simulink library "ctrl_ADRC_TD"  (R2018b)
settings: Solver=VariableStepAuto  StartTime=0.0  StopTime=10.0  RelTol=1e-3
settings Model: Creator=Huitao Lv  LastModifiedBy=Huitao Lv

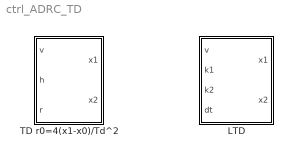
== system ctrl_ADRC_TD ==
  LTD : Subsystem  mask(LTD){}
      mask help: 线性跟踪微分器
  TD r0=4(x1-x0)/Td^2 : Subsystem  mask(TD){}
      mask help: 非线性跟踪微分器

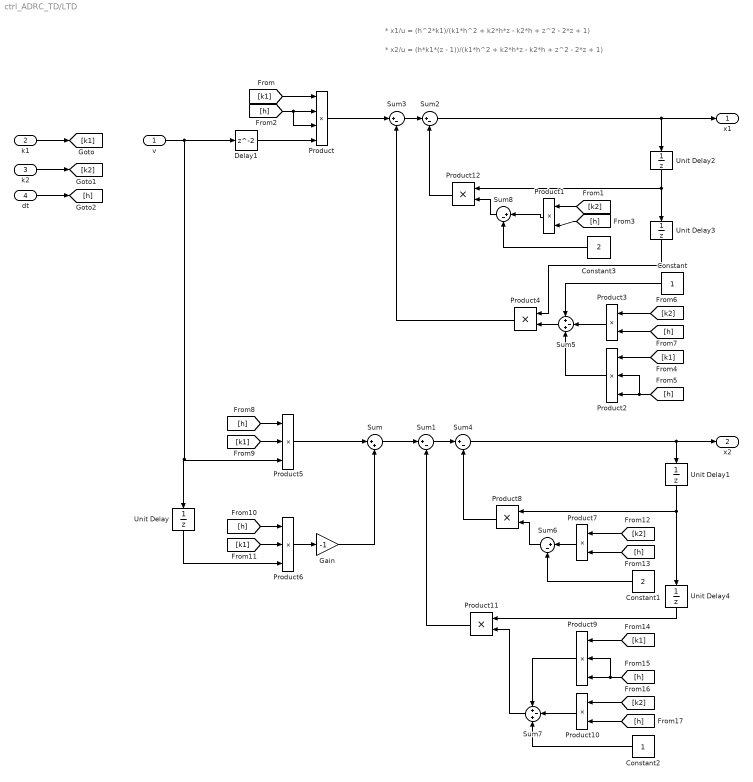
== system ctrl_ADRC_TD/LTD ==
  note: * x1/u = (h^2*k1)/(k1*h^2 + k2*h*z - k2*h + z^2 - 2*z + 1)
  note: * x2/u = (h*k1*(z - 1))/(k1*h^2 + k2*h*z - k2*h + z^2 - 2*z + 1)
  v : Inport
  k1 : Inport  Port=2
  k2 : Inport  Port=3
  dt : Inport  Port=4
  Constant : Constant  OutDataTypeStr=single
  Constant1 : Constant  Value=2  OutDataTypeStr=single
  Constant2 : Constant  OutDataTypeStr=single
  Constant3 : Constant  Value=2  OutDataTypeStr=single
  Delay1 : Delay
  Gain : Gain  Gain=-1
      settings: AttributesFormatString=%<Gain>
  Product : Product  Inputs=4
  Product1 : Product  Inputs=**
  Product{3..4,7..8,10..12} (7 alike) : Product
  Product{2,5..6,9} (4 alike) : Product  Inputs=3
  Sum : Sum  Inputs=|++
  Sum{1..4,6,8} (6 alike) : Sum  Inputs=|+-
  Sum5 : Sum  Inputs=+-+
  Sum7 : Sum  Inputs=+-+
  Unit Delay{,1..4} (5 alike) : UnitDelay  SampleTime=-1
  x1 : Outport
  x2 : Outport  Port=2
  wires:
  Constant3/1 -> Sum8/2
  Sum8/1 -> Product12/2
  Unit Delay2/1 -> Unit Delay3/1, Product12/1
  Product12/1 -> Sum2/2
  Product1/1 -> Sum8/1
  [k2] -> Product1/1
  Sum2/1 -> Unit Delay2/1, x1/1
  Unit Delay4/1 -> Product11/1
  Gain/1 -> Sum/2
  Product/1 -> Sum3/1
  Sum3/1 -> Sum2/1
  Unit Delay3/1 -> Product4/1
  Product8/1 -> Sum4/2
  Product4/1 -> Sum3/2
  v/1 -> Delay1/1, Product5/3, Unit Delay/1
  Unit Delay1/1 -> Unit Delay4/1, Product8/1
  Product5/1 -> Sum/1
  Sum/1 -> Sum1/1
  Delay1/1 -> Product/4
  Sum1/1 -> Sum4/1
  Sum4/1 -> x2/1, Unit Delay1/1
  Product11/1 -> Sum1/2
  dt/1 -> [h]
  k2/1 -> [k2]
  k1/1 -> [k1]
  [k1] -> Product/1
  [h] -> Product/3, Product/2
  [h] -> Product1/2
  [k1] -> Product2/1
  [h] -> Product2/2, Product2/3
  [k2] -> Product3/1
  [h] -> Product3/2
  Product2/1 -> Sum5/3
  Product3/1 -> Sum5/2
  Constant/1 -> Sum5/1
  Sum5/1 -> Product4/2
  [h] -> Product5/1
  [k1] -> Product5/2
  [k1] -> Product6/2
  [h] -> Product6/1
  Product6/1 -> Gain/1
  Unit Delay/1 -> Product6/3
  [k2] -> Product7/1
  [h] -> Product7/2
  Product7/1 -> Sum6/1
  Constant1/1 -> Sum6/2
  Sum6/1 -> Product8/2
  [h] -> Product9/3, Product9/2
  [k1] -> Product9/1
  Product9/1 -> Sum7/1
  Product10/1 -> Sum7/2
  [h] -> Product10/2
  [k2] -> Product10/1
  Constant2/1 -> Sum7/3
  Sum7/1 -> Product11/2

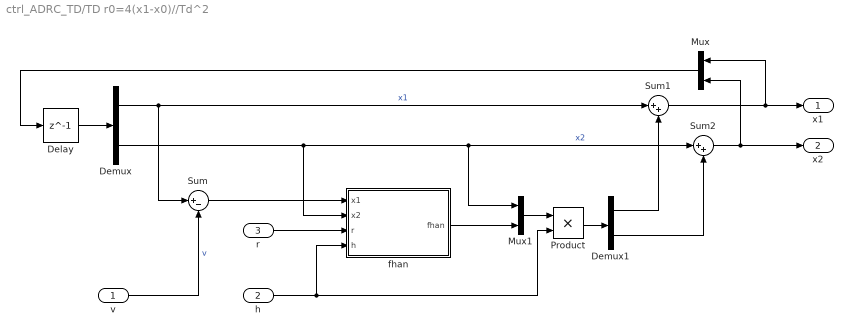
== system ctrl_ADRC_TD/TD r0=4(x1-x0)//Td^2 ==
  v : Inport
  h : Inport  Port=2
  r : Inport  Port=3
  Delay : Delay  DelayLength=1
  Demux : Demux  Outputs=2
  Demux1 : Demux  Outputs=2
  Mux : Mux  Inputs=2
  Mux1 : Mux  Inputs=2
  Product : Product
  Sum : Sum  Inputs=|+-
  Sum1 : Sum  Inputs=|++
  Sum2 : Sum  Inputs=|++
  fhan : Subsystem  mask(fhan){}
      mask help: 最优控制函数
  x1 : Outport
  x2 : Outport  Port=2
  wires:
  h/1 -> fhan/4(h), Product/2
  v/1 -> Sum/2  "v"
  Sum2/1 -> x2/1, Mux/2
  Sum1/1 -> x1/1, Mux/1
  Mux1/1 -> Product/1
  Demux1/2 -> Sum2/2
  fhan/1(fhan) -> Mux1/2
  Demux/1 -> Sum/1, Sum1/1  "x1"
  Demux1/1 -> Sum1/2
  Product/1 -> Demux1/1
  Mux/1 -> Delay/1
  Delay/1 -> Demux/1
  Demux/2 -> fhan/2(x2), Mux1/1, Sum2/1  "x2"
  Sum/1 -> fhan/1(x1)
  r/1 -> fhan/3(r)

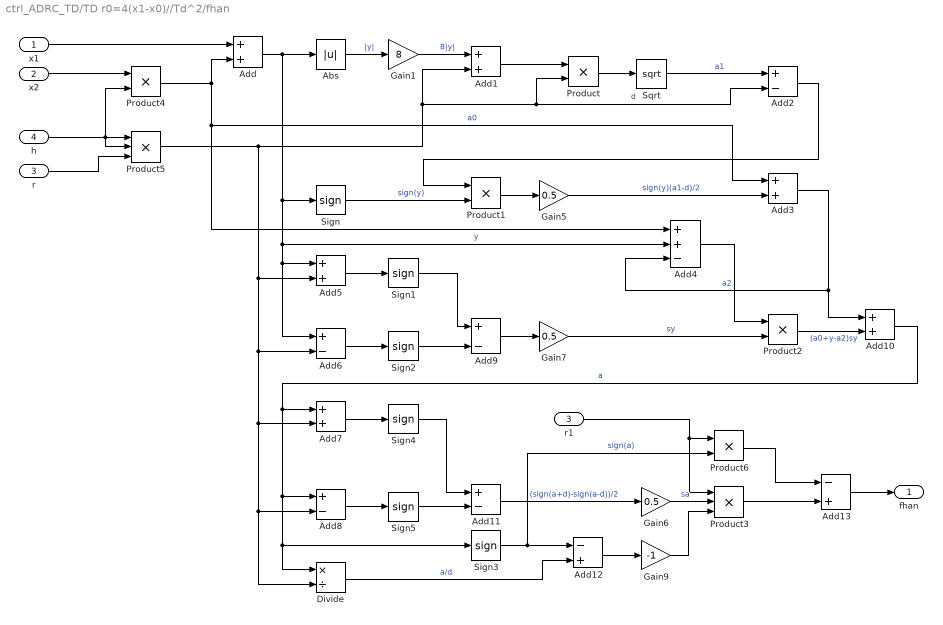
== system ctrl_ADRC_TD/TD r0=4(x1-x0)//Td^2/fhan ==
  x1 : Inport
  x2 : Inport  Port=2
  r : Inport  Port=3
  h : Inport  Port=4
  Abs : Abs
  Add{,1,3,5,7,10} (6 alike) : Sum
  Add{2,6,8..9,11} (5 alike) : Sum  Inputs=+-
  Add12 : Sum  Inputs=-+
  Add13 : Sum  Inputs=-+
  Add4 : Sum  Inputs=++-
  Divide : Product  Inputs=*/
  Gain1 : Gain  Gain=8
  Gain5 : Gain  Gain=0.5
  Gain6 : Gain  Gain=0.5
  Gain7 : Gain  Gain=0.5
  Gain9 : Gain  Gain=-1
  Product{,1..2,4,6} (5 alike) : Product
  Product3 : Product  Inputs=3
  Product5 : Product  Inputs=3
  Sign{,1..5} (6 alike) : Signum
  Sqrt : Sqrt  SaturateOnIntegerOverflow=on
  r1 : InportShadow  Port=3
  fhan : Outport
  wires:
  Sign4/1 -> Add11/1
  Product/1 -> Sqrt/1
  Add9/1 -> Gain7/1
  Add11/1 -> Gain6/1  "(sign(a+d)-sign(a-d))/2"
  Gain7/1 -> Product2/2  "sy"
  Add10/1 -> Add7/1, Add8/1, Sign3/1, Divide/1  "a"
  Product6/1 -> Add13/1
  Add6/1 -> Sign2/1
  Product1/1 -> Gain5/1
  Sign2/1 -> Add9/2
  Product3/1 -> Add13/2
  Add3/1 -> Add4/3, Add10/1  "a2"
  Product2/1 -> Add10/2  "(a0+y-a2)sy"
  Sign/1 -> Product1/2  "sign(y)"
  Gain5/1 -> Add3/2  "sign(y)(a1-d)/2"
  Sign1/1 -> Add9/1
  Add2/1 -> Product1/1
  Divide/1 -> Add12/2  "a/d"
  Sqrt/1 -> Add2/1  "a1"
  Add8/1 -> Sign5/1
  Abs/1 -> Gain1/1  "|y|"
  Gain1/1 -> Add1/1  "8|y|"
  Add12/1 -> Gain9/1
  Sign5/1 -> Add11/2
  Sign3/1 -> Product6/2, Add12/1  "sign(a)"
  Product5/1 -> Add5/2, Add6/2, Add7/2, Add8/2, Divide/2, Add1/2, Add2/2, Product/2  "d"
  x1/1 -> Add/1
  Product4/1 -> Add/2, Add3/1, Add4/1  "a0"
  Add13/1 -> fhan/1
  Gain6/1 -> Product3/2  "sa"
  Add/1 -> Abs/1, Add4/2, Add5/1, Add6/1, Sign/1  "y"
  Add5/1 -> Sign1/1
  Add7/1 -> Sign4/1
  Gain9/1 -> Product3/3
  x2/1 -> Product4/1
  Add4/1 -> Product2/1
  Add1/1 -> Product/1
  h/1 -> Product4/2, Product5/2, Product5/1
  r/1 -> Product5/3
  r1/1 -> Product6/1, Product3/1
